simulink model "trajectory_planner"  (R2019b)
settings: Solver=VariableStepAuto  StartTime=0.0  StopTime=10.0  RelTol=1e-3
libraries: robotcorelib x1
settings Model: Creator=logan  LastModifiedBy=logan
settings DataIOCC: ReturnWorkspaceOutputs=off
settings DebuggingCC: ArithmeticOperatorsInVariantConditions=warning
settings SFSimCC: CustomCodeUndefinedFunction=UseInterfaceOnly

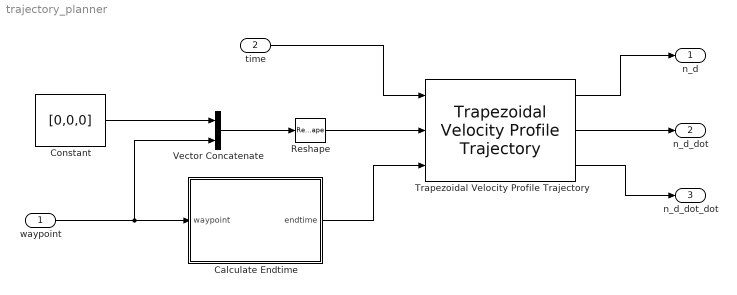
== system trajectory_planner ==
  "waypoint " : Inport
  "time " : Inport  Port=2
  Calculate Endtime : MATLAB Function  TreatAsAtomicUnit=on
  Constant : Constant  Value=[0,0,0]
  Reshape : Reshape  OutputDimensionality=Customize  OutputDimensions=[3,2]
  Trapezoidal Velocity Profile Trajectory : robotcorelib/Trapezoidal Velocity Profile Trajectory  WaypointSource=External  Waypoints=[ 0, -0.5, -1; 0, 0.5, 1 ]  NumParams=1  Parameter1=End Time  Parameter2=Peak Velocity  ParameterSource=External  PeakVelocity=[ 2; 2 ]  Acceleration=[ 1; 2 ]  EndTime=[ 1; 1 ]  AccelTime=[ 1; 2 ]  SimulateUsing=Interpreted execution
      settings: SourceProductName=Robotics System Toolbox  SourceProductBaseCode=RO
  Vector Concatenate : Concatenate
  n_d : Outport
  n_d_dot : Outport  Port=2
  n_d_dot_dot : Outport  Port=3
  wires:
  Trapezoidal Velocity Profile Trajectory/1 -> n_d/1
  Trapezoidal Velocity Profile Trajectory/2 -> n_d_dot/1
  Trapezoidal Velocity Profile Trajectory/3 -> n_d_dot_dot/1
  Calculate Endtime/1(endtime) -> Trapezoidal Velocity Profile Trajectory/3
  Reshape/1 -> Trapezoidal Velocity Profile Trajectory/2
  "waypoint "/1 -> Vector Concatenate/2, Calculate Endtime/1(waypoint)
  Vector Concatenate/1 -> Reshape/1
  Constant/1 -> Vector Concatenate/1
  "time "/1 -> Trapezoidal Velocity Profile Trajectory/1

== matlab function trajectory_planner/Calculate Endtime ==
  data: waypoint input; endtime output
function endtime = fcn(waypoint)

speed = 2;

endtime = sqrt(sum(waypoint .^ 2))/speed;
